simulink model "do_an_tn_ks"  (R2023b)
settings: Solver=VariableStepDiscrete  StartTime=0.0  StopTime=2  MaxStep=1e-7  RelTol=1e-3
values from neighbouring files (symbols this model uses):
  anpha = Vmax^3/(2*Ve*Vmax^2-2*Ve^3)    [daks_delay.m]
  b1 = 2-(wh*Ts1)^2    (= 1.99975325989)    [daks_delay.m]
  b2 = -1    [daks_delay.m]
  b3 = kprv1    [daks_delay.m]
  b4 = kirv1*Ts1+kprv1*((wh*Ts1)^2-2)    [daks_delay.m]
  b5 = kprv1-kirv1*Ts1    [daks_delay.m]
  C = Cmin    [daks_delay.m]
  c1 = 1    [daks_delay.m]
  c2 = kpi+kii*Ts/2    [daks_delay.m]
  c3 = kii*Ts/2-kpi    [daks_delay.m]
  Cf = 20e-6    (= 2e-05)    [daks_delay.m]
  ki1 = Ve/(sqrt(2)*Pe1)    [daks_delay.m]
  ki2 = Ve/(sqrt(2)*Pe2)    [daks_delay.m]
  kv = Vmax/sqrt(2)    [daks_delay.m]
  L = 1.3e-3    (= 0.0013)    [daks_delay.m]
  m4 = (4*m1/Ts^2+2*m2/Ts+m3)/(4*n1/Ts^2+2*n2/Ts+n3)    [daks_delay.m]
  m5 = (-8*m1/Ts^2+2*m3)/(4*n1/Ts^2+2*n2/Ts+n3)    [daks_delay.m]
  m6 = (4*m1/Ts^2-2*m2/Ts+m3)/(4*n1/Ts^2+2*n2/Ts+n3)    [daks_delay.m]
  n5 = -(-8*n1/Ts^2+2*n3)/(4*n1/Ts^2+2*n2/Ts+n3)    [daks_delay.m]
  n6 = -(4*n1/Ts^2-2*n2/Ts+n3)/(4*n1/Ts^2+2*n2/Ts+n3)    [daks_delay.m]
  o = 2*anpha    [daks_delay.m]
  Rf = 0.3    [daks_delay.m]
  sw = 4    [daks_delay.m]
  sw1 = 20    [daks_delay.m]
  Ts = 1/20000    (= 5e-05)    [daks_delay.m]
  Udc = 100    [daks_delay.m]
  wnom = 2*pi*50    (= 314.159265359)    [daks_delay.m]
undefined symbols (not defined in the file or in its folder): den_nz1, den_nz2, DiscIntNeverNeededParam, do_an_tn_ks, Down, i, m, num_nz1, num_nz2, Up
libraries: prociolib x12, peripheralslib x12, spsCurrentMeasurementLib x8, spsIGBTDiodeLib x8, spsSeriesRLCBranchLib x7, simulink x6, spsVoltageMeasurementLib x5, spsBreakerLib x2, simulink_extras x2, spsPowerLib x2, spsDCVoltageSourceLib x2, spsSeriesRLCLoadLib x1
(part 1 of 2)
settings Model: SimulationMode=accelerator  Creator=LEGION  LastModifiedBy=Acer
settings SolverCC: ZeroCrossControl=DisableAll  AlgebraicLoopSolver=TrustRegion
settings DataIOCC: ReturnWorkspaceOutputs=off
settings OptimizationCC: ReuseModelBlockBuffer=off
settings DebuggingCC: UnconnectedInputMsg=warning  UnconnectedOutputMsg=warning  UnconnectedLineMsg=warning
settings ModelReferenceCC: EnableRefExpFcnMdlSchedulingChecks=on
settings SFSimCC: CustomCodeUndefinedFunction=UseInterfaceOnly
settings GRTTargetCC: RTWCAPISignals=on  RTWCAPIParams=on

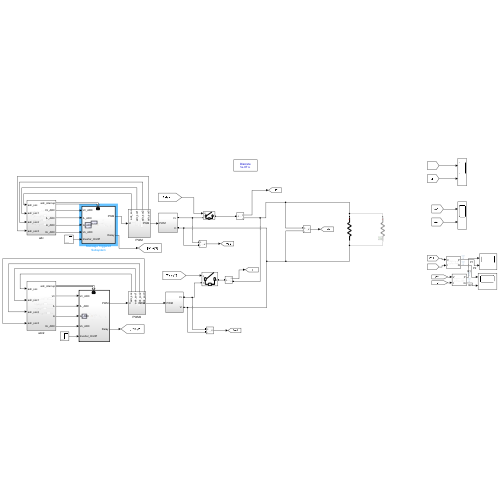
[thumbnail: Simulink's stored preview of the top-level diagram]
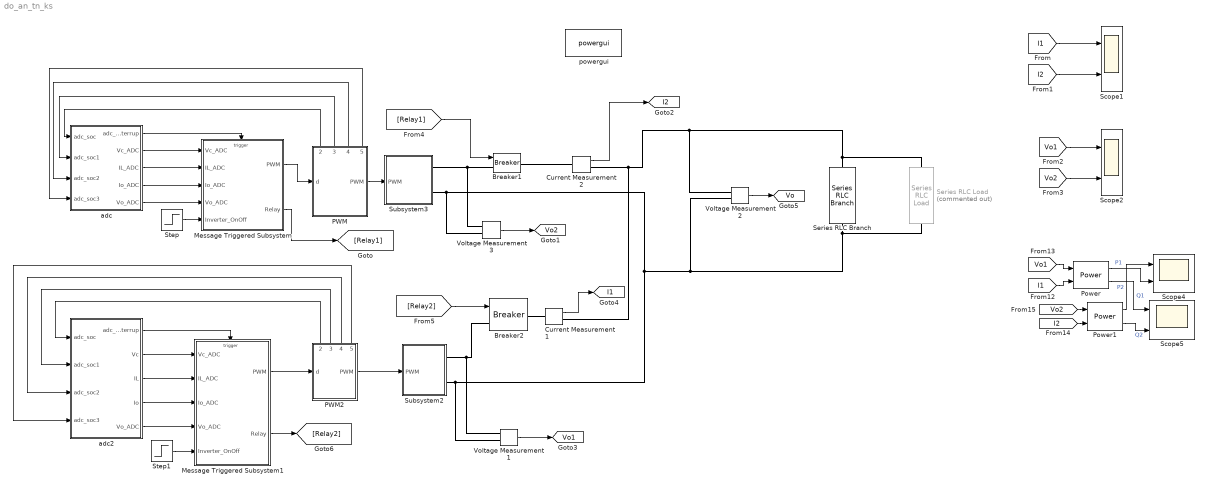
== system do_an_tn_ks ==
  Breaker1 : spsBreakerLib/Breaker  InitialState=0  SwitchingTimes="[1/60  5/60]"  External=on  BreakerResistance=0.01  SnubberResistance=1e6  SnubberCapacitance=inf  Measurements=None  MoreParameters=on  NoBreakLoop=off
  Breaker2 : spsBreakerLib/Breaker  InitialState=0  SwitchingTimes="[1/60  5/60]"  External=on  BreakerResistance=0.01  SnubberResistance=1e6  SnubberCapacitance=inf  Measurements=None  MoreParameters=on  NoBreakLoop=off
  Current Measurement1 : spsCurrentMeasurementLib/Current Measurement  PhasorSimulation=off  OutputType=Complex  PSBequivalent=0
  Current Measurement2 : spsCurrentMeasurementLib/Current Measurement  PhasorSimulation=off  OutputType=Complex  PSBequivalent=0
  Message Triggered Subsystem : Subsystem  InputPortMessageModes=i,i,i,i,i,m  TreatAsAtomicUnit=on
  Message Triggered Subsystem1 : Subsystem  InputPortMessageModes=i,i,i,i,i,m  TreatAsAtomicUnit=on
  PWM : Subsystem
      settings: PortSchema="{\"entries\":[{\"content\":{\"sides\":[{\"content\":{\"connectorIds\":[\"In1\"]},\"type\":\"ConnectorPlacement.EquallySpacedRectSide\",\"uuid\":\"e068b76d-8b58-4347-943a-c1dd0ef851be\"},{\"content\":{\"connectorIds\":[\"Out1\"],\"side\":\"RIGHT\"},\"type\":\"ConnectorPlacement.EquallySpacedRectSide\",\"uuid\":\"70af7750-8974-45f5-ac9e-e83d9d9c07fc\"},{\"content\":{\"connectorIds\":[\"Out2\",\"Out3\",\"Out4\",\"Out5\"],\"side\":\"TOP\"},\"type\":\"ConnectorPlacement.EquallySpacedRectSide\",\"uuid\":\"5d6a6e74-8176-4c49-8c99-236b0d61d046\"}]},\"type\":\"ConnectorPlacement.EquallySpacedConnector\",\"uuid\":\"483dab25-8052-4e69-8bb9-48464924440c\"}],\"packageUris\":[\"http://schema.mathworks.com/mf0/Connector/R2020b\"],\"version\":\"1.0\"}"
  PWM2 : Subsystem
      settings: PortSchema="{\"entries\":[{\"content\":{\"sides\":[{\"content\":{\"connectorIds\":[\"In1\"]},\"type\":\"ConnectorPlacement.EquallySpacedRectSide\",\"uuid\":\"e068b76d-8b58-4347-943a-c1dd0ef851be\"},{\"content\":{\"connectorIds\":[\"Out1\"],\"side\":\"RIGHT\"},\"type\":\"ConnectorPlacement.EquallySpacedRectSide\",\"uuid\":\"70af7750-8974-45f5-ac9e-e83d9d9c07fc\"},{\"content\":{\"connectorIds\":[\"Out2\",\"Out3\",\"Out4\",\"Out5\"],\"side\":\"TOP\"},\"type\":\"ConnectorPlacement.EquallySpacedRectSide\",\"uuid\":\"5d6a6e74-8176-4c49-8c99-236b0d61d046\"}]},\"type\":\"ConnectorPlacement.EquallySpacedConnector\",\"uuid\":\"483dab25-8052-4e69-8bb9-48464924440c\"}],\"packageUris\":[\"http://schema.mathworks.com/mf0/Connector/R2020b\"],\"version\":\"1.0\"}"
  Power : spsPowerLib/Power  Freq=50  Vinit=[1, 0]  Iinit=[1, 0]  Ts=Ts
  Power1 : spsPowerLib/Power  Freq=50  Vinit=[1, 0]  Iinit=[1, 0]  Ts=Ts
  Scope{1..2,4..5} (4 alike) : Scope  NumInputPorts=2
  Series RLC Branch : spsSeriesRLCBranchLib/Series RLC Branch  LConnTagsString=__new0  RConnTagsString=__new0  BranchType=R  Resistance=50  Inductance=1e-3  SetiL0=off  InitialCurrent=0  Capacitance=1e-6  Setx0=off  InitialVoltage=0  Measurements=None
  Series RLC Load : spsSeriesRLCLoadLib/Series RLC Load  Commented=on  LConnTagsString=a  RConnTagsString=__new0  NominalVoltage=220  NominalFrequency=50  ActivePower=3000  InductivePower=0  CapacitivePower=0  Setx0=off  InitialVoltage=0  SetiL0=off  InitialCurrent=0  Measurements=None  LoadType=constant Z
  Step : Step  Time=0.2  SampleTime=0
  Step1 : Step  Time=0.3  SampleTime=0
  Subsystem2 : Subsystem
  Subsystem3 : Subsystem
  Voltage Measurement1 : spsVoltageMeasurementLib/Voltage Measurement  PhasorSimulation=off  OutputType=Complex  PSBequivalent=0
  Voltage Measurement2 : spsVoltageMeasurementLib/Voltage Measurement  PhasorSimulation=off  OutputType=Complex  PSBequivalent=0
  Voltage Measurement3 : spsVoltageMeasurementLib/Voltage Measurement  PhasorSimulation=off  OutputType=Complex  PSBequivalent=0
  adc : Subsystem
  adc2 : Subsystem
  powergui : spspowerguiLib/powergui  Priority=1  SimulationMode=Discrete  SampleTime=1e-7  frequency=60  Iterations=50  frequencyindice=0  Pbase=100e6  ErrMax=1e-4  UnitsV=kV  UnitsW=MW  buscounter=0  FunctionMessages=off  echomessages=off  EnableUseOfTLC=off  CurrentSourceSwitches=off  DisableSnubberDevices=off  DisableRonSwitches=off  DisableVfSwitches=off  DisplayEquations=off  AutomaticDiscreteSolvers=off  SolverType=Tustin/Backward Euler (TBE)  Interpol=off  ExternalGateDelay=off  methode=off  Ts=100  x0status=blocks  SPID=on  SwTol=0  HookPort=off  NonlinearTolerance=1e-4  nMaxIteration=100  ContinueOnMaxIteration=off  RestoreLinks=warning  ResistiveCurrentMeasurement=off  Frange=[0:2:500]  Ylog=off  Xlog=on  ShowGrid=off  save=off  variable=ZData  structure=0  ZoomFFT=off  StartTime=0.0  cycles=1  DisplayStyle=1  fundamental=60  FreqAxis=off  MaxFrequency=1000  frequencyindicesteady=1  RmsSteady=1  display=off
  tag scope: I1=global, I2=global, Vo1=global, Vo2=global, Vo=global
  wires:
  adc/1(adc_interrup) -> Message Triggered Subsystem/Trigger
  PWM/1(PWM) -> Subsystem3/1("PWM ")
  adc/2(Vc_ADC) -> Message Triggered Subsystem/1(Vc_ADC)
  Message Triggered Subsystem/1(PWM) -> PWM/1(d)
  PWM/3(adc_soc1) -> adc/2(adc_soc1)
  PWM/2(adc_soc) -> adc/1(adc_soc)
  Voltage Measurement3/1 -> [Vo2]
  adc/3(IL_ADC) -> Message Triggered Subsystem/2(IL_ADC)
  PWM/4(adc_soc2) -> adc/3(adc_soc2)
  adc/4(Io_ADC) -> Message Triggered Subsystem/3(Io_ADC)
  Voltage Measurement1/1 -> [Vo1]
  PWM2/4(adc_soc2) -> adc2/3(adc_soc2)
  PWM2/2(adc_soc) -> adc2/1(adc_soc)
  PWM2/3(adc_soc1) -> adc2/2(adc_soc1)
  adc2/2(Vc) -> Message Triggered Subsystem1/1(Vc_ADC)
  PWM2/1(PWM) -> Subsystem2/1("PWM ")
  adc2/1(adc_interrup) -> Message Triggered Subsystem1/Trigger
  Current Measurement2/1 -> [I2]
  Current Measurement1/1 -> [I1]
  [I1] -> Scope1/1
  [I2] -> Scope1/2
  Step/1 -> Message Triggered Subsystem/5(Inverter_OnOff)
  [Vo1] -> Scope2/1
  [Vo2] -> Scope2/2
  Voltage Measurement2/1 -> [Vo]
  PWM/5(adc_soc3) -> adc/4(adc_soc3)
  adc/5(Vo_ADC) -> Message Triggered Subsystem/4(Vo_ADC)
  Power/1 -> Scope4/2  "P1"
  [Vo1] -> Power/1
  Power/2 -> Scope5/1  "Q1"
  Power1/2 -> Scope5/2  "Q2"
  [I2] -> Power1/2
  [I1] -> Power/2
  Power1/1 -> Scope4/1  "P2"
  [Vo2] -> Power1/1
  Message Triggered Subsystem1/1(PWM) -> PWM2/1(d)
  adc2/3(IL) -> Message Triggered Subsystem1/2(IL_ADC)
  adc2/4(Io) -> Message Triggered Subsystem1/3(Io_ADC)
  PWM2/5(adc_soc3) -> adc2/4(adc_soc3)
  adc2/5(Vo_ADC) -> Message Triggered Subsystem1/4(Vo_ADC)
  Step1/1 -> Message Triggered Subsystem1/5(Inverter_OnOff)
  Message Triggered Subsystem/2(Relay) -> [Relay1]
  [Relay1] -> Breaker1/1
  Message Triggered Subsystem1/2(Relay) -> [Relay2]
  [Relay2] -> Breaker2/1
  connections:
  Voltage Measurement3/LConn2 -- Subsystem3/RConn2 -- Series RLC Load/RConn1 -- Series RLC Branch/RConn1 -- Voltage Measurement2/LConn2 -- Voltage Measurement1/LConn2 -- Subsystem2/RConn2
  Breaker1/LConn1 -- Voltage Measurement3/LConn1 -- Subsystem3/RConn1
  Breaker1/RConn1 -- Current Measurement2/LConn1
  Current Measurement1/RConn1 -- Series RLC Branch/LConn1 -- Series RLC Load/LConn1 -- Voltage Measurement2/LConn1 -- Current Measurement2/RConn1
  Breaker2/RConn1 -- Current Measurement1/LConn1
  Breaker2/LConn1 -- Voltage Measurement1/LConn1 -- Subsystem2/RConn1

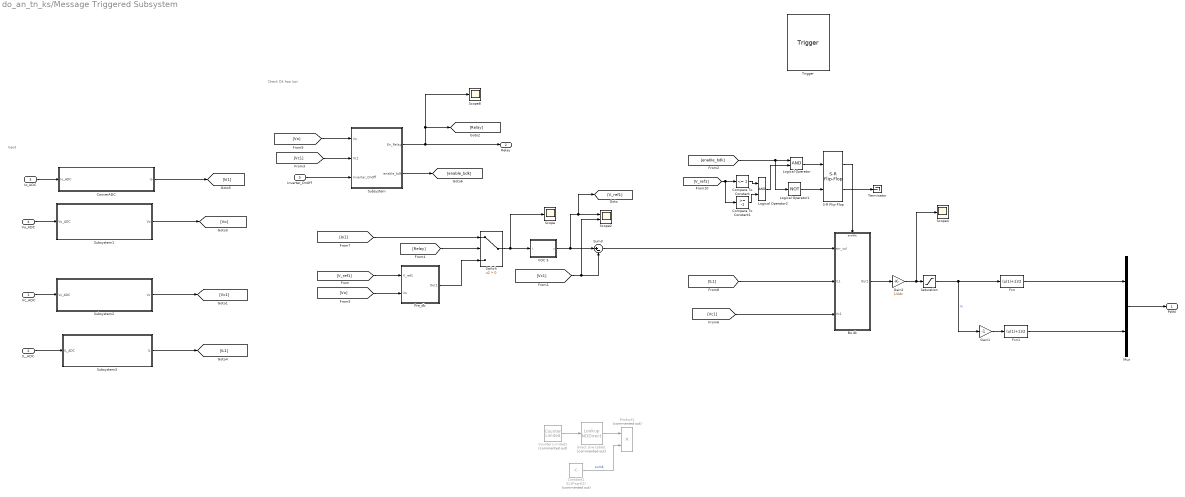
== system do_an_tn_ks/Message Triggered Subsystem ==
  note: Check Dk hoa luoi
  note: Input
  Vc_ADC : Inport
  IL_ADC : Inport  Port=2
  Io_ADC : Inport  Port=3
  Vo_ADC : Inport  Port=4
  Inverter_OnOff : Inport  Port=5
  Trigger : TriggerPort  TriggerType=message  ScheduleAsAperiodic=off  FunctionName=MessageTriggeredSubsystem  FunctionVisibility=scoped  VariantControl=(inherit)  PortDimensions=1
  Bo dk : Subsystem
  Compare To Constant : simulink/Logic and Bit Operations/Compare To Constant  relop=<=  const=1  OutDataTypeStr=boolean
  Compare To Constant1 : simulink/Logic and Bit Operations/Compare To Constant  relop=>=  const=-1  OutDataTypeStr=boolean
  Constant1 : Constant  Commented=on  Value=51.8*sqrt(2)  OutDataTypeStr=single  SampleTime=-1
  ConverADC : Subsystem
  Counter Limited1 : simulink/Sources/Counter Limited  Commented=on  uplimit=399  tsamp=-1
  Fcn : Fcn  Expr=(u(1)+1)/2
  Fcn1 : Fcn  Expr=(u(1)+1)/2
  Gain1 : Gain  Gain=-1
  Gain2 : Gain  Gain=1/Udc
  Logical Operator : Logic  AllPortsSameDT=off  OutDataTypeStr=boolean
  Logical Operator1 : Logic  Operator=NOT  AllPortsSameDT=off  OutDataTypeStr=boolean
  Logical Operator2 : Logic  AllPortsSameDT=off  OutDataTypeStr=boolean
  Mux : Mux  Inputs=2
  Pre_db : Subsystem
  Product1 : Product  Commented=on
  S-R Flip-Flop : simulink_extras/Flip Flops/S-R Flip-Flop  initial_condition=0
  Saturation : Saturate  UpperLimit=1  LowerLimit=-1
  Scope : Scope
  Scope2 : Scope  NumInputPorts=2
  Scope4 : Scope
  Scope8 : Scope
  Subsystem : Subsystem
  Subsystem1 : Subsystem
  Subsystem2 : Subsystem
  Subsystem3 : Subsystem
  Sum3 : Sum  Inputs=|+-
  Switch : Switch  Criteria=u2 > Threshold  SaturateOnIntegerOverflow=off  InputSameDT=off
  Terminator : Terminator
  VOC 3 : Subsystem
  direct sine table1 : LookupNDDirect  Commented=on  NumberOfTableDimensions=1  Table=sin( 2*pi *50* (0:399)/20000)'  TableDataTypeStr=single
  PWM : Outport
  Relay : Outport  Port=2
  wires:
  Constant1/1 -> Product1/2  "sum6"
  direct sine table1/1 -> Product1/1
  Sum3/1 -> Bo dk/1(err_vol)
  Saturation/1 -> Fcn/1, Gain1/1  "m"
  Gain1/1 -> Fcn1/1
  Gain2/1 -> Scope4/1, Saturation/1
  Counter Limited1/1 -> direct sine table1/1
  Mux/1 -> PWM/1
  Fcn/1 -> Mux/1
  Fcn1/1 -> Mux/2
  VOC 3/1(v) -> [V_ref1], Scope2/1, Sum3/1
  Switch/1 -> Scope/1, VOC 3/1(i)
  [Relay] -> Switch/2
  [Vc1] -> Scope2/2, Sum3/2
  [Vo] -> Subsystem/1(Vo)
  [Vc1] -> Subsystem/2(Vc1)
  Inverter_OnOff/1 -> Subsystem/3(Inverter_OnOff)
  Subsystem/1(En_Relay) -> Scope8/1, [Relay], Relay/1
  Io_ADC/1 -> ConverADC/1(Io_ADC)
  Subsystem1/1(Vo) -> [Vo]
  Vo_ADC/1 -> Subsystem1/1(Vo_ADC)
  Vc_ADC/1 -> Subsystem2/1(Vc_ADC)
  Subsystem2/1(Vc) -> [Vc1]
  IL_ADC/1 -> Subsystem3/1(IL_ADC)
  Subsystem3/1(IL) -> [IL1]
  [V_ref1] -> Pre_db/1(V_ref1)
  [Vo] -> Pre_db/2(Vo)
  Pre_db/1(Out1) -> Switch/3
  ConverADC/1(Io) -> [Io1]
  [Io1] -> Switch/1
  [IL1] -> Bo dk/2(IL1)
  [Vc1] -> Bo dk/3(Vc1)
  Bo dk/1(Out1) -> Gain2/1
  Subsystem/2(enable_bdk) -> [enable_bdk]
  Logical Operator1/1 -> S-R Flip-Flop/2
  S-R Flip-Flop/2 -> Terminator/1
  S-R Flip-Flop/1 -> Bo dk/Enable
  Logical Operator/1 -> S-R Flip-Flop/1
  [enable_bdk] -> Logical Operator1/1, Logical Operator/1
  [V_ref1] -> Compare To Constant1/1, Compare To Constant/1
  Compare To Constant/1 -> Logical Operator2/1
  Compare To Constant1/1 -> Logical Operator2/2
  Logical Operator2/1 -> Logical Operator/2

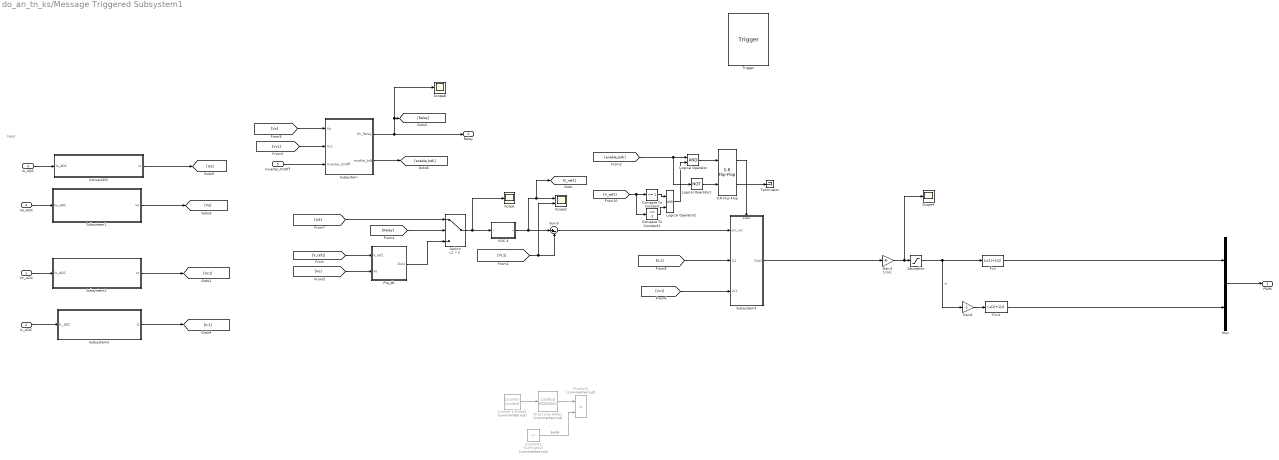
== system do_an_tn_ks/Message Triggered Subsystem1 ==
  note: Input
  Vc_ADC : Inport
  IL_ADC : Inport  Port=2
  Io_ADC : Inport  Port=3
  Vo_ADC : Inport  Port=4
  Inverter_OnOff : Inport  Port=5
  Trigger : TriggerPort  TriggerType=message  ScheduleAsAperiodic=off  FunctionName=MessageTriggeredSubsystem1  FunctionVisibility=scoped  VariantControl=(inherit)  PortDimensions=1
  Compare To Constant : simulink/Logic and Bit Operations/Compare To Constant  relop=<=  const=1  OutDataTypeStr=boolean
  Compare To Constant1 : simulink/Logic and Bit Operations/Compare To Constant  relop=>=  const=-1  OutDataTypeStr=boolean
  Constant1 : Constant  Commented=on  Value=51.8*sqrt(2)  OutDataTypeStr=single  SampleTime=-1
  ConverADC : Subsystem
  Counter Limited1 : simulink/Sources/Counter Limited  Commented=on  uplimit=399  tsamp=-1
  Fcn : Fcn  Expr=(u(1)+1)/2
  Fcn1 : Fcn  Expr=(u(1)+1)/2
  Gain1 : Gain  Gain=-1
  Gain2 : Gain  Gain=1/Udc
  Logical Operator : Logic  AllPortsSameDT=off  OutDataTypeStr=boolean
  Logical Operator1 : Logic  Operator=NOT  AllPortsSameDT=off  OutDataTypeStr=boolean
  Logical Operator2 : Logic  AllPortsSameDT=off  OutDataTypeStr=boolean
  Mux : Mux  Inputs=2
  Pre_db : Subsystem
  Product1 : Product  Commented=on
  S-R Flip-Flop : simulink_extras/Flip Flops/S-R Flip-Flop  initial_condition=0
  Saturation : Saturate  UpperLimit=1  LowerLimit=-1
  Scope : Scope
  Scope2 : Scope  NumInputPorts=2
  Scope4 : Scope
  Scope8 : Scope
  Subsystem : Subsystem
  Subsystem1 : Subsystem
  Subsystem2 : Subsystem
  Subsystem3 : Subsystem
  Subsystem4 : Subsystem
  Sum3 : Sum  Inputs=|+-
  Switch : Switch  Criteria=u2 > Threshold  SaturateOnIntegerOverflow=off  InputSameDT=off
  Terminator : Terminator
  VOC 3 : Subsystem
  direct sine table1 : LookupNDDirect  Commented=on  NumberOfTableDimensions=1  Table=sin( 2*pi *50* (0:399)/20000)'  TableDataTypeStr=single
  PWM : Outport
  Relay : Outport  Port=2
  wires:
  Subsystem/2(enable_bdk) -> [enable_bdk]
  Subsystem4/1(Out1) -> Gain2/1
  [Vc1] -> Subsystem4/3(Vc1)
  [IL1] -> Subsystem4/2(IL1)
  [Io1] -> Switch/1
  ConverADC/1(Io) -> [Io1]
  Pre_db/1(Out1) -> Switch/3
  [Vo] -> Pre_db/2(Vo)
  [V_ref1] -> Pre_db/1(V_ref1)
  Subsystem3/1(IL) -> [IL1]
  IL_ADC/1 -> Subsystem3/1(IL_ADC)
  Subsystem2/1(Vc) -> [Vc1]
  Vc_ADC/1 -> Subsystem2/1(Vc_ADC)
  Vo_ADC/1 -> Subsystem1/1(Vo_ADC)
  Subsystem1/1(Vo) -> [Vo]
  Io_ADC/1 -> ConverADC/1(Io_ADC)
  Subsystem/1(En_Relay) -> Relay/1, [Relay], Scope8/1
  Inverter_OnOff/1 -> Subsystem/3(Inverter_OnOff)
  [Vc1] -> Subsystem/2(Vc1)
  [Vo] -> Subsystem/1(Vo)
  [Vc1] -> Sum3/2, Scope2/2
  [Relay] -> Switch/2
  Switch/1 -> VOC 3/1(i), Scope/1
  VOC 3/1(v) -> Sum3/1, Scope2/1, [V_ref1]
  Fcn1/1 -> Mux/2
  Fcn/1 -> Mux/1
  Mux/1 -> PWM/1
  Counter Limited1/1 -> direct sine table1/1
  Gain2/1 -> Saturation/1, Scope4/1
  Gain1/1 -> Fcn1/1
  Saturation/1 -> Gain1/1, Fcn/1  "m"
  Sum3/1 -> Subsystem4/1(err_vol)
  direct sine table1/1 -> Product1/1
  Constant1/1 -> Product1/2  "sum6"
  [enable_bdk] -> Logical Operator1/1, Logical Operator/1
  Logical Operator2/1 -> Logical Operator/2
  Logical Operator/1 -> S-R Flip-Flop/1
  S-R Flip-Flop/1 -> Subsystem4/Enable
  Logical Operator1/1 -> S-R Flip-Flop/2
  S-R Flip-Flop/2 -> Terminator/1
  Compare To Constant1/1 -> Logical Operator2/2
  Compare To Constant/1 -> Logical Operator2/1
  [V_ref1] -> Compare To Constant1/1, Compare To Constant/1

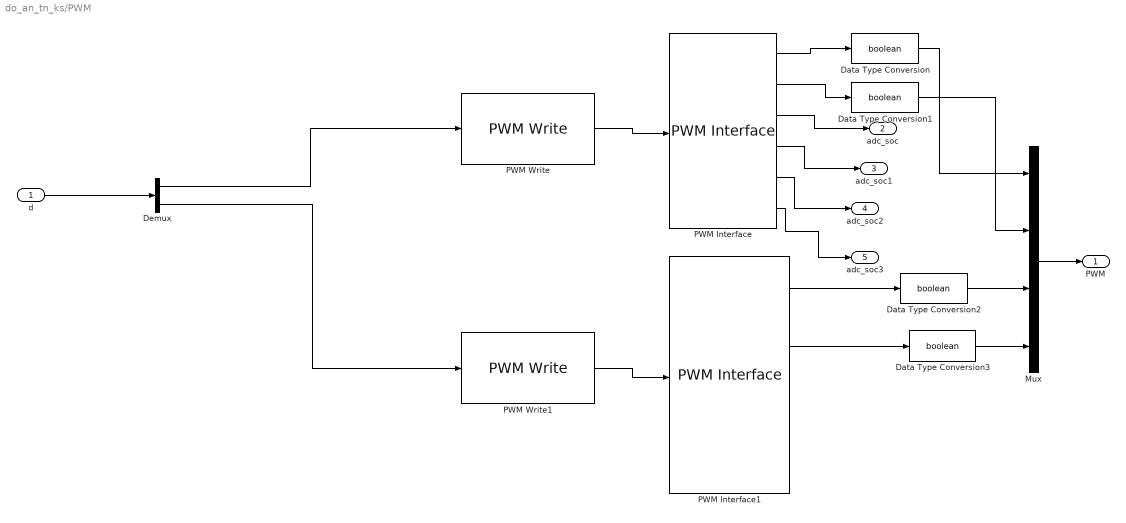
== system do_an_tn_ks/PWM ==
  d : Inport
  Data Type Conversion{,1..3} (4 alike) : DataTypeConversion  OutDataTypeStr=boolean  SaturateOnIntegerOverflow=off  RndMeth=Floor
  Demux : Demux  Outputs=2
  Mux : Mux
  PWM Interface : peripheralslib/PWM Interface  Period=1/10e3  OutSigMode=Switching  CounterMode=Up-Down  GenCompPWM=on  DeadTimeTopPWM=2e-6  DeadTimeBottomPWM=2e-6  EventCondition2=End of PWM period  DataType=single  PWMAtStartPeriod=High  PWMAtMidPeriod=NoChange  PWMAtCMP1=Low  PWMAtCMP1UpCnt=Low  PWMAtCMP1DwnCnt=High  PWMAtCMP2=NoChange  PWMAtCMP2UpCnt=NoChange  PWMAtCMP2DwnCnt=NoChange  OutCountDir=off  PhaseOffset=0  EventType=ADC start  EventCondition1=Mid or End of PWM period  NumADCSOCToWait=1st event  NumADCSOCReplica=4  InterruptCond=End of PWM period  IntLatency=0  NumInterruptToWait=1st event
      settings: SamplingMode=Mid or End of PWM period
  PWM Interface1 : peripheralslib/PWM Interface  Period=1/10e3  OutSigMode=Switching  CounterMode=Up-Down  GenCompPWM=on  DeadTimeTopPWM=2e-6  DeadTimeBottomPWM=2e-6  EventCondition2=End of PWM period  DataType=single  PWMAtStartPeriod=High  PWMAtMidPeriod=NoChange  PWMAtCMP1=Low  PWMAtCMP1UpCnt=Low  PWMAtCMP1DwnCnt=High  PWMAtCMP2=NoChange  PWMAtCMP2UpCnt=NoChange  PWMAtCMP2DwnCnt=NoChange  OutCountDir=off  PhaseOffset=0  EventType=ADC start  EventCondition1=Mid of PWM period  NumADCSOCToWait=1st event  NumADCSOCReplica=2  InterruptCond=End of PWM period  IntLatency=0  NumInterruptToWait=1st event
      settings: SamplingMode=Mid or End of PWM period
  PWM Write : prociolib/PWM Write  ShowPeriodInp=off  ShowPhaseInp=off  PeripheralConfigBtnCtrl=0  BlockSID=do_an_tn_ks:3474
  PWM Write1 : prociolib/PWM Write  ShowPeriodInp=off  ShowPhaseInp=off  PeripheralConfigBtnCtrl=0  BlockSID=do_an_tn_ks:3475
  PWM : Outport
  adc_soc : Outport  Port=2
  adc_soc1 : Outport  Port=3
  adc_soc2 : Outport  Port=4
  adc_soc3 : Outport  Port=5
  wires:
  PWM Write1/1 -> PWM Interface1/1
  Data Type Conversion1/1 -> Mux/2
  PWM Write/1 -> PWM Interface/1
  PWM Interface/2 -> Data Type Conversion1/1
  Mux/1 -> PWM/1
  Demux/2 -> PWM Write1/1
  PWM Interface/1 -> Data Type Conversion/1
  Data Type Conversion2/1 -> Mux/3
  Data Type Conversion3/1 -> Mux/4
  PWM Interface1/2 -> Data Type Conversion3/1
  Data Type Conversion/1 -> Mux/1
  PWM Interface1/1 -> Data Type Conversion2/1
  Demux/1 -> PWM Write/1
  d/1 -> Demux/1
  PWM Interface/3 -> adc_soc/1
  PWM Interface/4 -> adc_soc1/1
  PWM Interface/5 -> adc_soc2/1
  PWM Interface/6 -> adc_soc3/1

== system do_an_tn_ks/PWM2 ==
  d : Inport
  Data Type Conversion{,1..3} (4 alike) : DataTypeConversion  OutDataTypeStr=boolean  SaturateOnIntegerOverflow=off  RndMeth=Floor
  Demux : Demux  Outputs=2
  Mux : Mux
  PWM Interface : peripheralslib/PWM Interface  Period=1/10e3  OutSigMode=Switching  CounterMode=Up-Down  GenCompPWM=on  DeadTimeTopPWM=2e-6  DeadTimeBottomPWM=2e-6  EventCondition2=End of PWM period  DataType=single  PWMAtStartPeriod=High  PWMAtMidPeriod=NoChange  PWMAtCMP1=Low  PWMAtCMP1UpCnt=Low  PWMAtCMP1DwnCnt=High  PWMAtCMP2=NoChange  PWMAtCMP2UpCnt=NoChange  PWMAtCMP2DwnCnt=NoChange  OutCountDir=off  PhaseOffset=0  EventType=ADC start  EventCondition1=Mid or End of PWM period  NumADCSOCToWait=1st event  NumADCSOCReplica=4  InterruptCond=End of PWM period  IntLatency=0  NumInterruptToWait=1st event
      settings: SamplingMode=Mid or End of PWM period
  PWM Interface1 : peripheralslib/PWM Interface  Period=1/10e3  OutSigMode=Switching  CounterMode=Up-Down  GenCompPWM=on  DeadTimeTopPWM=2e-6  DeadTimeBottomPWM=2e-6  EventCondition2=End of PWM period  DataType=single  PWMAtStartPeriod=High  PWMAtMidPeriod=NoChange  PWMAtCMP1=Low  PWMAtCMP1UpCnt=Low  PWMAtCMP1DwnCnt=High  PWMAtCMP2=NoChange  PWMAtCMP2UpCnt=NoChange  PWMAtCMP2DwnCnt=NoChange  OutCountDir=off  PhaseOffset=0  EventType=ADC start  EventCondition1=Mid of PWM period  NumADCSOCToWait=1st event  NumADCSOCReplica=2  InterruptCond=End of PWM period  IntLatency=0  NumInterruptToWait=1st event
      settings: SamplingMode=Mid or End of PWM period
  PWM Write : prociolib/PWM Write  ShowPeriodInp=off  ShowPhaseInp=off  PeripheralConfigBtnCtrl=0  BlockSID=do_an_tn_ks:3847
  PWM Write1 : prociolib/PWM Write  ShowPeriodInp=off  ShowPhaseInp=off  PeripheralConfigBtnCtrl=0  BlockSID=do_an_tn_ks:3848
  PWM : Outport
  adc_soc : Outport  Port=2
  adc_soc1 : Outport  Port=3
  adc_soc2 : Outport  Port=4
  adc_soc3 : Outport  Port=5
  wires:
  PWM Interface/5 -> adc_soc2/1
  PWM Interface/4 -> adc_soc1/1
  PWM Interface/3 -> adc_soc/1
  d/1 -> Demux/1
  Demux/1 -> PWM Write/1
  PWM Interface1/1 -> Data Type Conversion2/1
  Data Type Conversion/1 -> Mux/1
  PWM Interface1/2 -> Data Type Conversion3/1
  Data Type Conversion3/1 -> Mux/4
  Data Type Conversion2/1 -> Mux/3
  PWM Interface/1 -> Data Type Conversion/1
  Demux/2 -> PWM Write1/1
  Mux/1 -> PWM/1
  PWM Interface/2 -> Data Type Conversion1/1
  PWM Write/1 -> PWM Interface/1
  Data Type Conversion1/1 -> Mux/2
  PWM Write1/1 -> PWM Interface1/1
  PWM Interface/6 -> adc_soc3/1

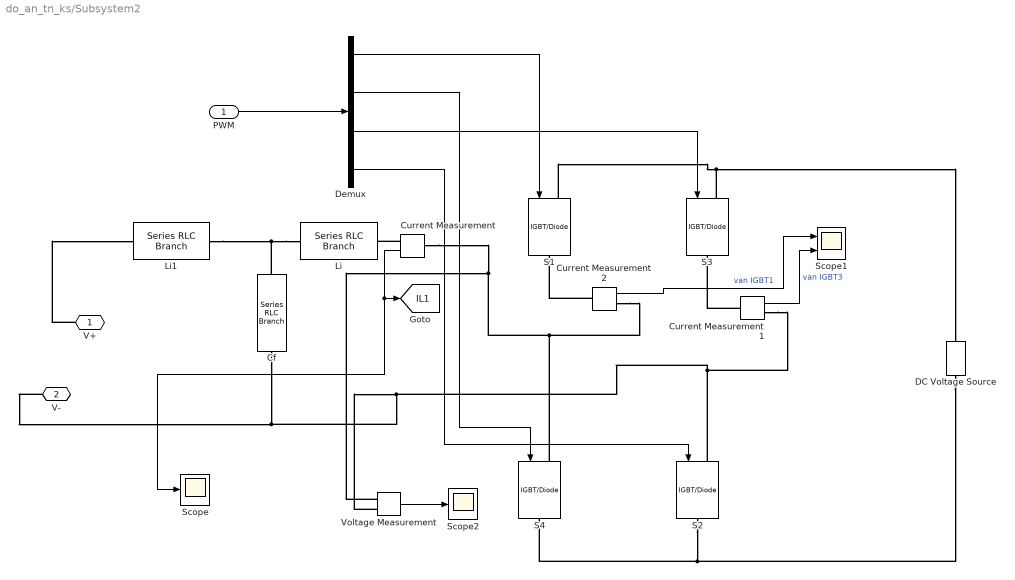
== system do_an_tn_ks/Subsystem2 ==
  "PWM " : Inport
  "   Cf" : spsSeriesRLCBranchLib/Series RLC Branch  LConnTagsString=__new0  RConnTagsString=__new0  BranchType=C  Resistance=0.1  Inductance=1e-3  SetiL0=off  InitialCurrent=0  Capacitance=Cf  Setx0=off  InitialVoltage=0  Measurements=None
  Current Measurement : spsCurrentMeasurementLib/Current Measurement  PhasorSimulation=off  OutputType=Complex  PSBequivalent=0
  Current Measurement1 : spsCurrentMeasurementLib/Current Measurement  PhasorSimulation=off  OutputType=Complex  PSBequivalent=0
  Current Measurement2 : spsCurrentMeasurementLib/Current Measurement  PhasorSimulation=off  OutputType=Complex  PSBequivalent=0
  DC Voltage Source : spsDCVoltageSourceLib/DC Voltage Source  Amplitude=Udc  Measurements=None
  Demux : Demux
  Li : spsSeriesRLCBranchLib/Series RLC Branch  LConnTagsString=__new0  RConnTagsString=__new0  BranchType=RL  Resistance=Rf  Inductance=L  SetiL0=off  InitialCurrent=0  Capacitance=1e-6  Setx0=off  InitialVoltage=0  Measurements=None
  Li1 : spsSeriesRLCBranchLib/Series RLC Branch  LConnTagsString=__new0  RConnTagsString=__new0  BranchType=L  Resistance=Rf  Inductance=470e-6  SetiL0=off  InitialCurrent=0  Capacitance=1e-6  Setx0=off  InitialVoltage=0  Measurements=None
  S{1..4} (4 alike) : spsIGBTDiodeLib/IGBT//Diode  Ron=0.001  Rs=1e5  Cs=inf  Measurements=off
  Scope : Scope
  Scope1 : Scope  NumInputPorts=2
  Scope2 : Scope
  Voltage Measurement : spsVoltageMeasurementLib/Voltage Measurement  PhasorSimulation=off  OutputType=Complex  PSBequivalent=0
  V+ : PMIOPort  Side=Right
  V- : PMIOPort  Port=2  Side=Right
  tag scope: IL1=global
  wires:
  Demux/4 -> S2/1
  Demux/3 -> S3/1
  Demux/2 -> S4/1
  Current Measurement2/1 -> Scope1/1  "van IGBT1"
  Voltage Measurement/1 -> Scope2/1
  Current Measurement1/1 -> Scope1/2  "van IGBT3"
  Current Measurement/1 -> [IL1], Scope/1
  Demux/1 -> S1/1
  "PWM "/1 -> Demux/1
  connections:
  Current Measurement2/LConn1 -- S1/RConn1
  Current Measurement1/LConn1 -- S3/RConn1
  Current Measurement/RConn1 -- Li/RConn1
  S4/RConn1 -- DC Voltage Source/LConn1 -- S2/RConn1
  "   Cf"/RConn1 -- V-/RConn1 -- Voltage Measurement/LConn2 -- Current Measurement1/RConn1 -- S2/LConn1
  S3/LConn1 -- S1/LConn1 -- DC Voltage Source/RConn1
  Current Measurement/LConn1 -- Voltage Measurement/LConn1 -- Current Measurement2/RConn1 -- S4/LConn1
  Li/LConn1 -- Li1/RConn1 -- "   Cf"/LConn1
  V+/RConn1 -- Li1/LConn1

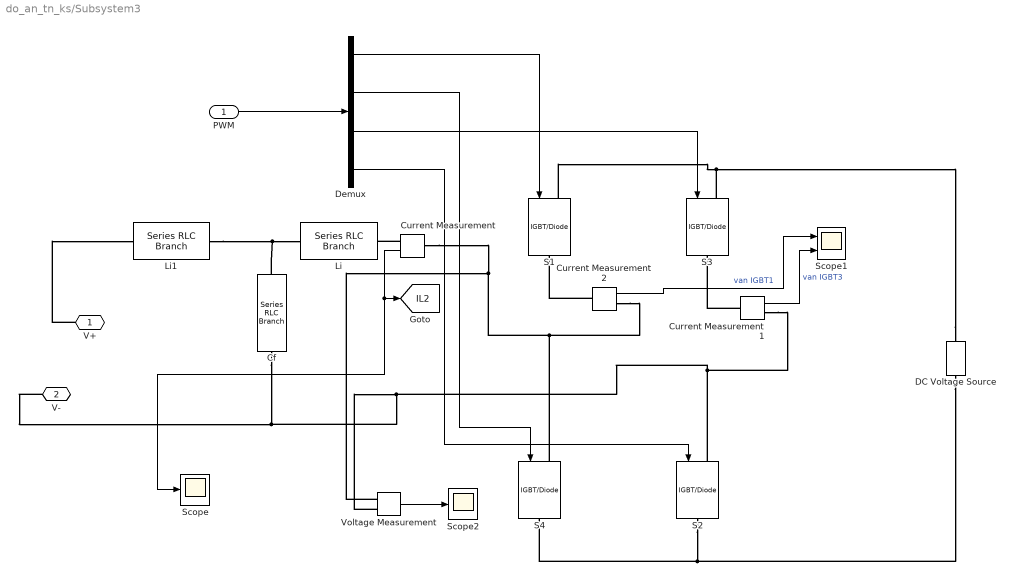
== system do_an_tn_ks/Subsystem3 ==
  "PWM " : Inport
  "   Cf" : spsSeriesRLCBranchLib/Series RLC Branch  LConnTagsString=__new0  RConnTagsString=__new0  BranchType=C  Resistance=0.1  Inductance=1e-3  SetiL0=off  InitialCurrent=0  Capacitance=Cf  Setx0=off  InitialVoltage=0  Measurements=None
  Current Measurement : spsCurrentMeasurementLib/Current Measurement  PhasorSimulation=off  OutputType=Complex  PSBequivalent=0
  Current Measurement1 : spsCurrentMeasurementLib/Current Measurement  PhasorSimulation=off  OutputType=Complex  PSBequivalent=0
  Current Measurement2 : spsCurrentMeasurementLib/Current Measurement  PhasorSimulation=off  OutputType=Complex  PSBequivalent=0
  DC Voltage Source : spsDCVoltageSourceLib/DC Voltage Source  Amplitude=Udc  Measurements=None
  Demux : Demux
  Li : spsSeriesRLCBranchLib/Series RLC Branch  LConnTagsString=__new0  RConnTagsString=__new0  BranchType=RL  Resistance=Rf  Inductance=L  SetiL0=off  InitialCurrent=0  Capacitance=1e-6  Setx0=off  InitialVoltage=0  Measurements=None
  Li1 : spsSeriesRLCBranchLib/Series RLC Branch  LConnTagsString=__new0  RConnTagsString=__new0  BranchType=L  Resistance=Rf  Inductance=470e-6  SetiL0=off  InitialCurrent=0  Capacitance=1e-6  Setx0=off  InitialVoltage=0  Measurements=None
  S{1..4} (4 alike) : spsIGBTDiodeLib/IGBT//Diode  Ron=0.001  Rs=1e5  Cs=inf  Measurements=off
  Scope : Scope
  Scope1 : Scope  NumInputPorts=2
  Scope2 : Scope
  Voltage Measurement : spsVoltageMeasurementLib/Voltage Measurement  PhasorSimulation=off  OutputType=Complex  PSBequivalent=0
  V+ : PMIOPort  Side=Right
  V- : PMIOPort  Port=2  Side=Right
  tag scope: IL2=global
  wires:
  "PWM "/1 -> Demux/1
  Demux/1 -> S1/1
  Current Measurement/1 -> Scope/1, [IL2]
  Current Measurement1/1 -> Scope1/2  "van IGBT3"
  Voltage Measurement/1 -> Scope2/1
  Current Measurement2/1 -> Scope1/1  "van IGBT1"
  Demux/2 -> S4/1
  Demux/3 -> S3/1
  Demux/4 -> S2/1
  connections:
  V+/RConn1 -- Li1/LConn1
  S4/LConn1 -- Current Measurement2/RConn1 -- Voltage Measurement/LConn1 -- Current Measurement/LConn1
  DC Voltage Source/RConn1 -- S1/LConn1 -- S3/LConn1
  S2/LConn1 -- Current Measurement1/RConn1 -- Voltage Measurement/LConn2 -- V-/RConn1 -- "   Cf"/RConn1
  S2/RConn1 -- DC Voltage Source/LConn1 -- S4/RConn1
  Current Measurement/RConn1 -- Li/RConn1
  Current Measurement1/LConn1 -- S3/RConn1
  Current Measurement2/LConn1 -- S1/RConn1
  Li1/RConn1 -- "   Cf"/LConn1 -- Li/LConn1

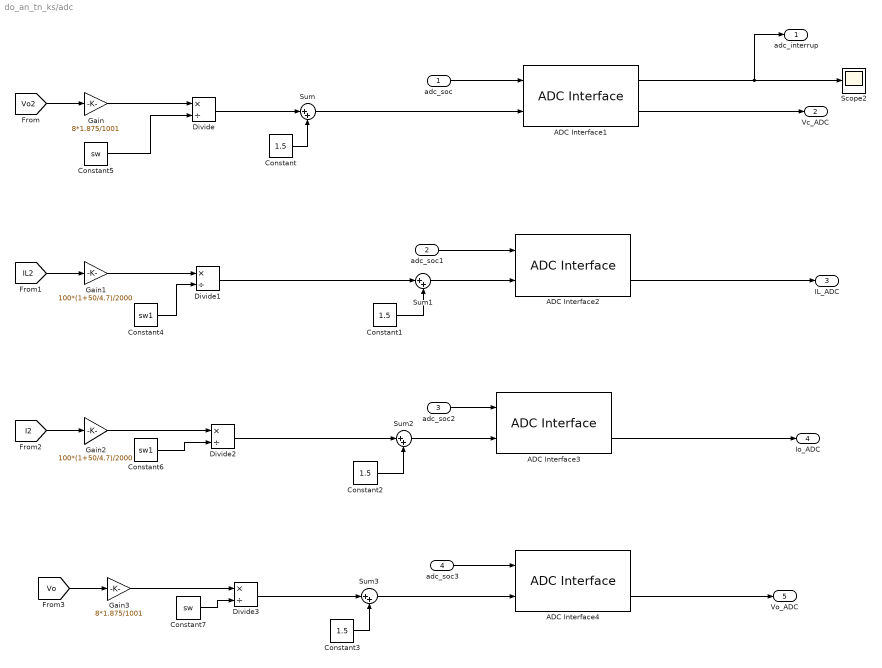
== system do_an_tn_ks/adc ==
  adc_soc : Inport
  adc_soc1 : Inport  Port=2
  adc_soc2 : Inport  Port=3
  adc_soc3 : Inport  Port=4
  ADC Interface{1..4} (4 alike) : peripheralslib/ADC Interface  ADCResolution=12  HighVref=3.3  AcqTime=15*1/(40e6)  ConvTime=12*1/(40e6)  TimeConstant=0  SoftTrig=off  SampleTime=1e-3  NumCh=1  ConvType=Sequential  EnInterrupt=on  IntCondition=Acquisition + Conversion time  EnWatchdog=off  LowThreshold=.1  HighThreshold=2.9  IntLatency=0
  Constant{,1..3} (4 alike) : Constant  Value=1.5
  Constant4 : Constant  Value=sw1
  Constant5 : Constant  Value=sw
  Constant6 : Constant  Value=sw1
  Constant7 : Constant  Value=sw
  Divide{,1..3} (4 alike) : Product  Inputs=*/
  Gain : Gain  Gain=8*1.875/1001
  Gain1 : Gain  Gain=100*(1+50/4.7)/2000
  Gain2 : Gain  Gain=100*(1+50/4.7)/2000
  Gain3 : Gain  Gain=8*1.875/1001
  Scope2 : Scope
  Sum{,1..3} (4 alike) : Sum  Inputs=|++
  adc_interrup : Outport
  Vc_ADC : Outport  Port=2
  IL_ADC : Outport  Port=3
  Io_ADC : Outport  Port=4
  Vo_ADC : Outport  Port=5
  wires:
  adc_soc/1 -> ADC Interface1/1
  [Vo2] -> Gain/1
  Constant/1 -> Sum/2
  Sum/1 -> ADC Interface1/2
  ADC Interface1/2 -> Vc_ADC/1
  adc_soc1/1 -> ADC Interface2/1
  [IL2] -> Gain1/1
  Sum1/1 -> ADC Interface2/2
  Constant1/1 -> Sum1/2
  ADC Interface1/1 -> adc_interrup/1, Scope2/1
  ADC Interface2/2 -> IL_ADC/1
  [I2] -> Gain2/1
  Constant2/1 -> Sum2/2
  ADC Interface3/2 -> Io_ADC/1
  adc_soc2/1 -> ADC Interface3/1
  Sum2/1 -> ADC Interface3/2
  Constant3/1 -> Sum3/2
  [Vo] -> Gain3/1
  adc_soc3/1 -> ADC Interface4/1
  Sum3/1 -> ADC Interface4/2
  ADC Interface4/2 -> Vo_ADC/1
  Gain/1 -> Divide/1
  Divide/1 -> Sum/1
  Gain1/1 -> Divide1/1
  Divide1/1 -> Sum1/1
  Divide2/1 -> Sum2/1
  Gain2/1 -> Divide2/1
  Gain3/1 -> Divide3/1
  Divide3/1 -> Sum3/1
  Constant5/1 -> Divide/2
  Constant4/1 -> Divide1/2
  Constant6/1 -> Divide2/2
  Constant7/1 -> Divide3/2

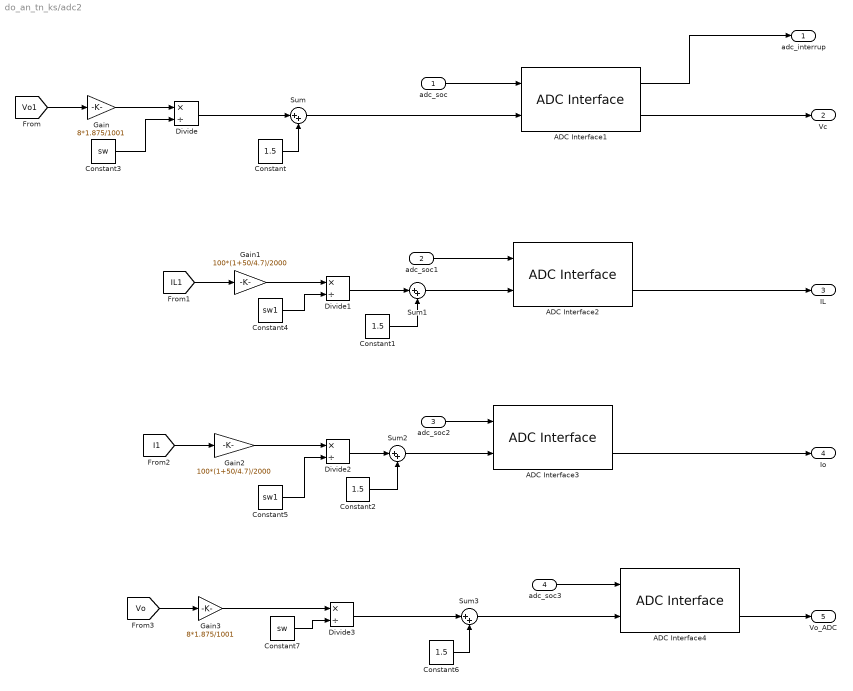
== system do_an_tn_ks/adc2 ==
  adc_soc : Inport
  adc_soc1 : Inport  Port=2
  adc_soc2 : Inport  Port=3
  adc_soc3 : Inport  Port=4
  ADC Interface{1..4} (4 alike) : peripheralslib/ADC Interface  ADCResolution=12  HighVref=3.3  AcqTime=15*1/(40e6)  ConvTime=12*1/(40e6)  TimeConstant=0  SoftTrig=off  SampleTime=1e-3  NumCh=1  ConvType=Sequential  EnInterrupt=on  IntCondition=Acquisition + Conversion time  EnWatchdog=off  LowThreshold=.1  HighThreshold=2.9  IntLatency=0
  Constant{,1..2,6} (4 alike) : Constant  Value=1.5
  Constant3 : Constant  Value=sw
  Constant4 : Constant  Value=sw1
  Constant5 : Constant  Value=sw1
  Constant7 : Constant  Value=sw
  Divide{,1..3} (4 alike) : Product  Inputs=*/
  Gain : Gain  Gain=8*1.875/1001
  Gain1 : Gain  Gain=100*(1+50/4.7)/2000
  Gain2 : Gain  Gain=100*(1+50/4.7)/2000
  Gain3 : Gain  Gain=8*1.875/1001
  Sum{,1..3} (4 alike) : Sum  Inputs=|++
  adc_interrup : Outport
  Vc : Outport  Port=2
  IL : Outport  Port=3
  Io : Outport  Port=4
  Vo_ADC : Outport  Port=5
  wires:
  Sum2/1 -> ADC Interface3/2
  adc_soc2/1 -> ADC Interface3/1
  ADC Interface3/2 -> Io/1
  Constant2/1 -> Sum2/2
  [I1] -> Gain2/1
  ADC Interface2/2 -> IL/1
  ADC Interface1/1 -> adc_interrup/1
  Constant1/1 -> Sum1/2
  Sum1/1 -> ADC Interface2/2
  [IL1] -> Gain1/1
  adc_soc1/1 -> ADC Interface2/1
  ADC Interface1/2 -> Vc/1
  Sum/1 -> ADC Interface1/2
  Constant/1 -> Sum/2
  [Vo1] -> Gain/1
  adc_soc/1 -> ADC Interface1/1
  Gain/1 -> Divide/1
  Gain1/1 -> Divide1/1
  Gain2/1 -> Divide2/1
  Divide2/1 -> Sum2/1
  Divide/1 -> Sum/1
  Divide1/1 -> Sum1/1
  Constant3/1 -> Divide/2
  Constant4/1 -> Divide1/2
  Constant5/1 -> Divide2/2
  Constant7/1 -> Divide3/2
  Constant6/1 -> Sum3/2
  Gain3/1 -> Divide3/1
  Divide3/1 -> Sum3/1
  ADC Interface4/2 -> Vo_ADC/1
  [Vo] -> Gain3/1
  adc_soc3/1 -> ADC Interface4/1
  Sum3/1 -> ADC Interface4/2

== system do_an_tn_ks/Message Triggered Subsystem/Bo dk ==
  err_vol : Inport
  IL1 : Inport  Port=2
  Vc1 : Inport  Port=3
  Enable : EnablePort
  Scope3 : Scope  NumInputPorts=2
  Sum : Sum  Inputs=|++
  Sum5 : Sum  Inputs=|+-
  curr_controller : Subsystem
  voltage_controller : Subsystem
  Out1 : Outport
  wires:
  Vc1/1 -> Sum/2
  Sum5/1 -> curr_controller/1(In1)
  curr_controller/1(Out1) -> Sum/1
  Sum/1 -> Out1/1
  err_vol/1 -> voltage_controller/1(In1)
  IL1/1 -> Scope3/2, Sum5/2
  voltage_controller/1(Out1) -> Scope3/1, Sum5/1

== system do_an_tn_ks/Message Triggered Subsystem/ConverADC ==
  Io_ADC : Inport
  Constant2 : Constant  Value=1.5*4096/3.3
  Constant9 : Constant  Value=sw1
  Current ADC Read - ADCC2 : prociolib/ADC Read  DataType=uint16  SampleTime=-1  NumCh=1  PeripheralConfigBtnCtrl=0  BlockSID=do_an_tn_ks:3536
  Data Type Conversion2 : DataTypeConversion  OutDataTypeStr=double  SaturateOnIntegerOverflow=off  RndMeth=Floor
  Gain3 : Gain  Gain=3.3*20/(4096*(1+50/4.7))
  Product : Product
  Sum1 : Sum  Inputs=|+-
  Io : Outport
  wires:
  Current ADC Read - ADCC2/1 -> Data Type Conversion2/1  "I_fbk"
  Data Type Conversion2/1 -> Sum1/1
  Constant9/1 -> Product/2
  Gain3/1 -> Product/1
  Constant2/1 -> Sum1/2
  Io_ADC/1 -> Current ADC Read - ADCC2/1
  Product/1 -> Io/1
  Sum1/1 -> Gain3/1

== system do_an_tn_ks/Message Triggered Subsystem/Pre_db ==
  V_ref1 : Inport
  Vo : Inport  Port=2
  Add : Sum  Inputs=+-
  Constant4 : Constant  Value=10
  Divide : Product  Inputs=*/
  Out1 : Outport
  wires:
  Add/1 -> Divide/1
  Vo/1 -> Add/2
  Constant4/1 -> Divide/2
  Divide/1 -> Out1/1
  V_ref1/1 -> Add/1

== system do_an_tn_ks/Message Triggered Subsystem/Subsystem ==
  Vo : Inport
  Vc1 : Inport  Port=2
  Inverter_OnOff : Inport  Port=3
  Abs : Abs  SaturateOnIntegerOverflow=off
  Abs1 : Abs  SaturateOnIntegerOverflow=off
  Chart1 : Stateflow chart  TreatAsAtomicUnit=on
      settings: PortSchema="{\"entries\":[{\"content\":{\"sides\":[{\"content\":{\"connectorIds\":[\"In4\",\"In3\",\"In1\",\"In2\"]},\"type\":\"ConnectorPlacement.EquallySpacedRectSide\",\"uuid\":\"a41d96ef-4339-445d-adf1-46a375c1ebfc\"},{\"content\":{\"connectorIds\":[\"Out1\",\"Out2\"],\"side\":\"RIGHT\"},\"type\":\"ConnectorPlacement.EquallySpacedRectSide\",\"uuid\":\"433b8e1f-da11-4860-b5b3-686501ffdddb\"},{\"content\":{\"side\":\"TOP\"},\"type\":\"ConnectorPlacement.EquallySpacedRectSide\",\"uuid\":\"a76241af-ec7f-4a92-ba0a-9793b7afdcf0\"}]},\"type\":\"ConnectorPlacement.EquallySpacedConnector\",\"uuid\":\"1de099f0-7c57-4924-8764-8a627297889a\"}],\"packageUris\":[\"http://schema.mathworks.com/mf0/Connector/R2020b\"],\"version\":\"1.0\"}"
  MATLAB Function : MATLAB Function  TreatAsAtomicUnit=on
  MATLAB Function1 : MATLAB Function  TreatAsAtomicUnit=on
  Scope6 : Scope
  Sum6 : Sum  Inputs=|+-
  Terminator : Terminator
  Terminator1 : Terminator
  En_Relay : Outport
  enable_bdk : Outport  Port=2
  wires:
  MATLAB Function/1(Vrms) -> Chart1/3(Vout_Rms), Sum6/1
  MATLAB Function1/2(theta) -> Terminator/1
  MATLAB Function/2(theta) -> Terminator1/1
  MATLAB Function1/1(Vrms) -> Sum6/2
  Abs1/1 -> Chart1/1(Error_RMS)
  Vc1/1 -> Abs/1, MATLAB Function1/1(vin)
  Sum6/1 -> Abs1/1, Scope6/1
  Abs/1 -> Chart1/4(Vc1_abs)
  Inverter_OnOff/1 -> Chart1/2(Inverter_OnOff)
  Chart1/1(En_Relay) -> En_Relay/1
  Vo/1 -> MATLAB Function/1(vin)
  Chart1/2(enable_bdk) -> enable_bdk/1

== system do_an_tn_ks/Message Triggered Subsystem/Subsystem1 ==
  Vo_ADC : Inport
  Constant5 : Constant  Value=1.5*4096/3.3
  Constant6 : Constant  Value=sw
  Current ADC Read - ADCC3 : prociolib/ADC Read  DataType=uint16  SampleTime=-1  NumCh=1  PeripheralConfigBtnCtrl=0  BlockSID=do_an_tn_ks:3953
  Data Type Conversion3 : DataTypeConversion  OutDataTypeStr=double  SaturateOnIntegerOverflow=off  RndMeth=Floor
  Gain4 : Gain  Gain=3.3*1001/(8*4096*1.875)
  Product2 : Product
  Sum8 : Sum  Inputs=|+-
  Vo : Outport
  wires:
  Sum8/1 -> Gain4/1
  Constant5/1 -> Sum8/2
  Current ADC Read - ADCC3/1 -> Data Type Conversion3/1  "I_fbk"
  Gain4/1 -> Product2/1
  Product2/1 -> Vo/1
  Data Type Conversion3/1 -> Sum8/1
  Vo_ADC/1 -> Current ADC Read - ADCC3/1
  Constant6/1 -> Product2/2

== system do_an_tn_ks/Message Triggered Subsystem/Subsystem2 ==
  Vc_ADC : Inport
  Constant : Constant  Value=1.5*4096/3.3
  Constant7 : Constant  Value=sw
  Current ADC Read - ADCC5 : prociolib/ADC Read  DataType=uint16  SampleTime=-1  NumCh=1  PeripheralConfigBtnCtrl=0  BlockSID=do_an_tn_ks:3404
  Data Type Conversion : DataTypeConversion  OutDataTypeStr=double  SaturateOnIntegerOverflow=off  RndMeth=Floor
  Gain13 : Gain  Gain=3.3*1001/(8*4096*1.875)
  Product3 : Product
  Sum2 : Sum  Inputs=|+-
  Vc : Outport
  wires:
  Gain13/1 -> Product3/1
  Current ADC Read - ADCC5/1 -> Data Type Conversion/1  "I_fbk"
  Sum2/1 -> Gain13/1
  Product3/1 -> Vc/1
  Constant/1 -> Sum2/2
  Vc_ADC/1 -> Current ADC Read - ADCC5/1
  Data Type Conversion/1 -> Sum2/1
  Constant7/1 -> Product3/2

== system do_an_tn_ks/Message Triggered Subsystem/Subsystem3 ==
  IL_ADC : Inport
  Constant3 : Constant  Value=1.5*4096/3.3
  Constant8 : Constant  Value=sw1
  Current ADC Read - ADCC1 : prociolib/ADC Read  DataType=uint16  SampleTime=-1  NumCh=1  PeripheralConfigBtnCtrl=0  BlockSID=do_an_tn_ks:3403
  Data Type Conversion1 : DataTypeConversion  OutDataTypeStr=double  SaturateOnIntegerOverflow=off  RndMeth=Floor
  Gain14 : Gain  Gain=3.3*20/(4096*(1+50/4.7))
  Product4 : Product
  Sum4 : Sum  Inputs=|+-
  IL : Outport
  wires:
  Current ADC Read - ADCC1/1 -> Data Type Conversion1/1  "I_fbk"
  Product4/1 -> IL/1
  Gain14/1 -> Product4/1
  Sum4/1 -> Gain14/1
  Constant3/1 -> Sum4/2
  Data Type Conversion1/1 -> Sum4/1
  Constant8/1 -> Product4/2
  IL_ADC/1 -> Current ADC Read - ADCC1/1

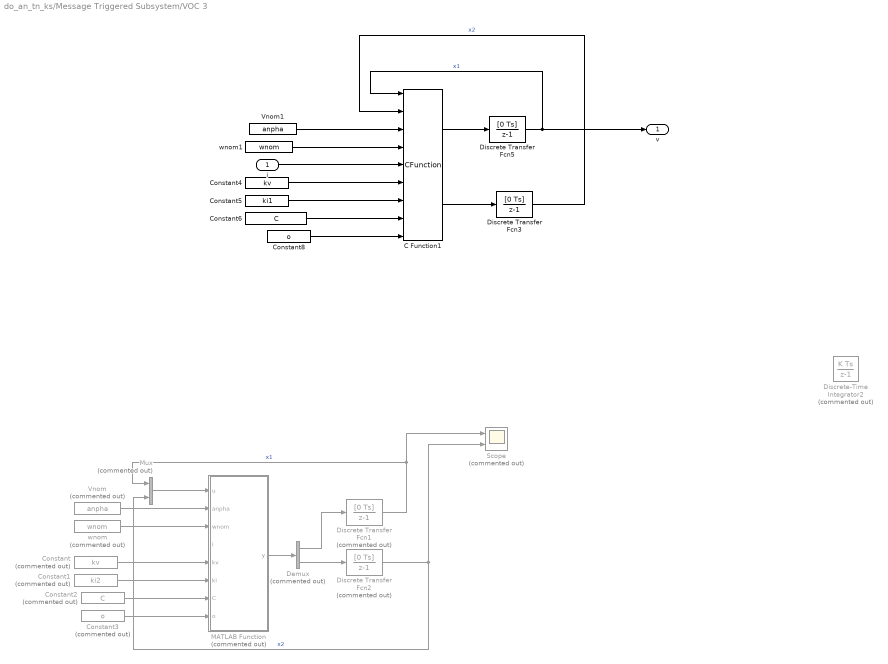
== system do_an_tn_ks/Message Triggered Subsystem/VOC 3 ==
  i : Inport
  C Function1 : CFunction  OutputCode=|
      | y1 = (kv*kv*o/anpha-u1*u1-u2*u2)*u1*anpha/(C*kv*kv)-wnom*u2-ki*kv*i/C;
      | y2 = wnom*u1;
  Constant : Constant  Commented=on  Value=kv  OutDataTypeStr=double  SampleTime=-1
  Constant1 : Constant  Commented=on  Value=ki2  OutDataTypeStr=double  SampleTime=-1
  Constant2 : Constant  Commented=on  Value=C  OutDataTypeStr=double  SampleTime=-1
  Constant3 : Constant  Commented=on  Value=o  OutDataTypeStr=double  SampleTime=-1
  Constant4 : Constant  Value=kv  OutDataTypeStr=double  SampleTime=-1
  Constant5 : Constant  Value=ki1  OutDataTypeStr=double  SampleTime=-1
  Constant6 : Constant  Value=C  OutDataTypeStr=double  SampleTime=-1
  Constant8 : Constant  Value=o  OutDataTypeStr=double  SampleTime=-1
  Demux : Demux  Commented=on  Outputs=2
  Discrete Transfer Fcn1 : DiscreteTransferFcn  Commented=on  Numerator=[0 Ts]  Denominator=[1 -1]  SampleTime=Ts
  Discrete Transfer Fcn2 : DiscreteTransferFcn  Commented=on  Numerator=[0 Ts]  Denominator=[1 -1]  SampleTime=Ts
  Discrete Transfer Fcn3 : DiscreteTransferFcn  Numerator=[0 Ts]  Denominator=[1 -1]
  Discrete Transfer Fcn5 : DiscreteTransferFcn  Numerator=[0 Ts]  Denominator=[1 -1]
  Discrete-Time Integrator2 : DiscreteIntegrator  Commented=on  InitialCondition=0.5  SampleTime=Ts  ICPrevOutput=DiscIntNeverNeededParam  ICPrevScaledInput=DiscIntNeverNeededParam
  MATLAB Function : MATLAB Function  Commented=on  TreatAsAtomicUnit=on
  Mux : Mux  Commented=on  Inputs=2
  Scope : Scope  Commented=on  NumInputPorts=2
  Vnom : Constant  Commented=on  Value=anpha  OutDataTypeStr=double  SampleTime=-1
  Vnom1 : Constant  Value=anpha  OutDataTypeStr=double  SampleTime=-1
  wnom : Constant  Commented=on  Value=wnom  OutDataTypeStr=double  SampleTime=-1
  wnom1 : Constant  Value=wnom  OutDataTypeStr=double  SampleTime=-1
  v : Outport
  wires:
  wnom/1 -> MATLAB Function/3(wnom)
  Discrete Transfer Fcn1/1 -> Scope/1, Mux/1  "x1"
  Mux/1 -> MATLAB Function/1(u)
  Demux/2 -> Discrete Transfer Fcn2/1
  MATLAB Function/1(y) -> Demux/1
  Demux/1 -> Discrete Transfer Fcn1/1
  Discrete Transfer Fcn2/1 -> Scope/2, Mux/2  "x2"
  Vnom/1 -> MATLAB Function/2(anpha)
  Constant/1 -> MATLAB Function/5(kv)
  Constant1/1 -> MATLAB Function/6(ki)
  Constant2/1 -> MATLAB Function/7(C)
  Constant3/1 -> MATLAB Function/8(o)
  Discrete Transfer Fcn5/1 -> C Function1/1, v/1  "x1"
  C Function1/1 -> Discrete Transfer Fcn5/1
  Vnom1/1 -> C Function1/3
  Constant8/1 -> C Function1/9
  Constant4/1 -> C Function1/6
  Constant6/1 -> C Function1/8
  C Function1/2 -> Discrete Transfer Fcn3/1
  wnom1/1 -> C Function1/4
  Constant5/1 -> C Function1/7
  Discrete Transfer Fcn3/1 -> C Function1/2  "x2"
  i/1 -> C Function1/5

== system do_an_tn_ks/Message Triggered Subsystem1/ConverADC ==
  Io_ADC : Inport
  Constant2 : Constant  Value=1.5*4096/3.3
  Constant9 : Constant  Value=sw1
  Current ADC Read - ADCC2 : prociolib/ADC Read  DataType=uint16  SampleTime=-1  NumCh=1  PeripheralConfigBtnCtrl=0  BlockSID=do_an_tn_ks:4141
  Data Type Conversion2 : DataTypeConversion  OutDataTypeStr=double  SaturateOnIntegerOverflow=off  RndMeth=Floor
  Gain3 : Gain  Gain=3.3*20/(4096*(1+50/4.7))
  Product : Product
  Sum1 : Sum  Inputs=|+-
  Io : Outport
  wires:
  Sum1/1 -> Gain3/1
  Product/1 -> Io/1
  Io_ADC/1 -> Current ADC Read - ADCC2/1
  Constant2/1 -> Sum1/2
  Gain3/1 -> Product/1
  Constant9/1 -> Product/2
  Data Type Conversion2/1 -> Sum1/1
  Current ADC Read - ADCC2/1 -> Data Type Conversion2/1  "I_fbk"

== system do_an_tn_ks/Message Triggered Subsystem1/Pre_db ==
  V_ref1 : Inport
  Vo : Inport  Port=2
  Add : Sum  Inputs=+-
  Constant4 : Constant  Value=10
  Divide : Product  Inputs=*/
  Out1 : Outport
  wires:
  V_ref1/1 -> Add/1
  Divide/1 -> Out1/1
  Constant4/1 -> Divide/2
  Vo/1 -> Add/2
  Add/1 -> Divide/1

== system do_an_tn_ks/Message Triggered Subsystem1/Subsystem ==
  Vo : Inport
  Vc1 : Inport  Port=2
  Inverter_OnOff : Inport  Port=3
  Abs : Abs  SaturateOnIntegerOverflow=off
  Abs1 : Abs  SaturateOnIntegerOverflow=off
  Chart1 : Stateflow chart  TreatAsAtomicUnit=on
      settings: PortSchema="{\"entries\":[{\"content\":{\"sides\":[{\"content\":{\"connectorIds\":[\"In4\",\"In3\",\"In1\",\"In2\"]},\"type\":\"ConnectorPlacement.EquallySpacedRectSide\",\"uuid\":\"a41d96ef-4339-445d-adf1-46a375c1ebfc\"},{\"content\":{\"connectorIds\":[\"Out1\",\"Out2\"],\"side\":\"RIGHT\"},\"type\":\"ConnectorPlacement.EquallySpacedRectSide\",\"uuid\":\"433b8e1f-da11-4860-b5b3-686501ffdddb\"},{\"content\":{\"side\":\"TOP\"},\"type\":\"ConnectorPlacement.EquallySpacedRectSide\",\"uuid\":\"a76241af-ec7f-4a92-ba0a-9793b7afdcf0\"}]},\"type\":\"ConnectorPlacement.EquallySpacedConnector\",\"uuid\":\"1de099f0-7c57-4924-8764-8a627297889a\"}],\"packageUris\":[\"http://schema.mathworks.com/mf0/Connector/R2020b\"],\"version\":\"1.0\"}"
  MATLAB Function : MATLAB Function  TreatAsAtomicUnit=on
  MATLAB Function1 : MATLAB Function  TreatAsAtomicUnit=on
  Scope6 : Scope
  Sum6 : Sum  Inputs=|+-
  Terminator : Terminator
  Terminator1 : Terminator
  En_Relay : Outport
  enable_bdk : Outport  Port=2
  wires:
  Chart1/2(enable_bdk) -> enable_bdk/1
  Vo/1 -> MATLAB Function/1(vin)
  Chart1/1(En_Relay) -> En_Relay/1
  Inverter_OnOff/1 -> Chart1/2(Inverter_OnOff)
  Abs/1 -> Chart1/4(Vc1_abs)
  Sum6/1 -> Scope6/1, Abs1/1
  Vc1/1 -> MATLAB Function1/1(vin), Abs/1
  Abs1/1 -> Chart1/1(Error_RMS)
  MATLAB Function1/1(Vrms) -> Sum6/2
  MATLAB Function/2(theta) -> Terminator1/1
  MATLAB Function1/2(theta) -> Terminator/1
  MATLAB Function/1(Vrms) -> Sum6/1, Chart1/3(Vout_Rms)

== system do_an_tn_ks/Message Triggered Subsystem1/Subsystem1 ==
  Vo_ADC : Inport
  Constant5 : Constant  Value=1.5*4096/3.3
  Constant6 : Constant  Value=sw
  Current ADC Read - ADCC3 : prociolib/ADC Read  DataType=uint16  SampleTime=-1  NumCh=1  PeripheralConfigBtnCtrl=0  BlockSID=do_an_tn_ks:4202
  Data Type Conversion3 : DataTypeConversion  OutDataTypeStr=double  SaturateOnIntegerOverflow=off  RndMeth=Floor
  Gain4 : Gain  Gain=3.3*1001/(8*4096*1.875)
  Product2 : Product
  Sum8 : Sum  Inputs=|+-
  Vo : Outport
  wires:
  Constant6/1 -> Product2/2
  Vo_ADC/1 -> Current ADC Read - ADCC3/1
  Data Type Conversion3/1 -> Sum8/1
  Product2/1 -> Vo/1
  Gain4/1 -> Product2/1
  Current ADC Read - ADCC3/1 -> Data Type Conversion3/1  "I_fbk"
  Constant5/1 -> Sum8/2
  Sum8/1 -> Gain4/1

== system do_an_tn_ks/Message Triggered Subsystem1/Subsystem2 ==
  Vc_ADC : Inport
  Constant : Constant  Value=1.5*4096/3.3
  Constant7 : Constant  Value=sw
  Current ADC Read - ADCC5 : prociolib/ADC Read  DataType=uint16  SampleTime=-1  NumCh=1  PeripheralConfigBtnCtrl=0  BlockSID=do_an_tn_ks:4212
  Data Type Conversion : DataTypeConversion  OutDataTypeStr=double  SaturateOnIntegerOverflow=off  RndMeth=Floor
  Gain13 : Gain  Gain=3.3*1001/(8*4096*1.875)
  Product3 : Product
  Sum2 : Sum  Inputs=|+-
  Vc : Outport
  wires:
  Constant7/1 -> Product3/2
  Data Type Conversion/1 -> Sum2/1
  Vc_ADC/1 -> Current ADC Read - ADCC5/1
  Constant/1 -> Sum2/2
  Product3/1 -> Vc/1
  Sum2/1 -> Gain13/1
  Current ADC Read - ADCC5/1 -> Data Type Conversion/1  "I_fbk"
  Gain13/1 -> Product3/1

== system do_an_tn_ks/Message Triggered Subsystem1/Subsystem3 ==
  IL_ADC : Inport
  Constant3 : Constant  Value=1.5*4096/3.3
  Constant8 : Constant  Value=sw1
  Current ADC Read - ADCC1 : prociolib/ADC Read  DataType=uint16  SampleTime=-1  NumCh=1  PeripheralConfigBtnCtrl=0  BlockSID=do_an_tn_ks:4222
  Data Type Conversion1 : DataTypeConversion  OutDataTypeStr=double  SaturateOnIntegerOverflow=off  RndMeth=Floor
  Gain14 : Gain  Gain=3.3*20/(4096*(1+50/4.7))
  Product4 : Product
  Sum4 : Sum  Inputs=|+-
  IL : Outport
  wires:
  IL_ADC/1 -> Current ADC Read - ADCC1/1
  Constant8/1 -> Product4/2
  Data Type Conversion1/1 -> Sum4/1
  Constant3/1 -> Sum4/2
  Sum4/1 -> Gain14/1
  Gain14/1 -> Product4/1
  Product4/1 -> IL/1
  Current ADC Read - ADCC1/1 -> Data Type Conversion1/1  "I_fbk"

== system do_an_tn_ks/Message Triggered Subsystem1/Subsystem4 ==
  err_vol : Inport
  IL1 : Inport  Port=2
  Vc1 : Inport  Port=3
  Enable : EnablePort
  Scope3 : Scope  NumInputPorts=2
  Sum : Sum  Inputs=|++
  Sum5 : Sum  Inputs=|+-
  curr_controller : Subsystem
  voltage_controller : Subsystem
  Out1 : Outport
  wires:
  voltage_controller/1(Out1) -> Sum5/1, Scope3/1
  IL1/1 -> Sum5/2, Scope3/2
  err_vol/1 -> voltage_controller/1(In1)
  Sum/1 -> Out1/1
  curr_controller/1(Out1) -> Sum/1
  Sum5/1 -> curr_controller/1(In1)
  Vc1/1 -> Sum/2

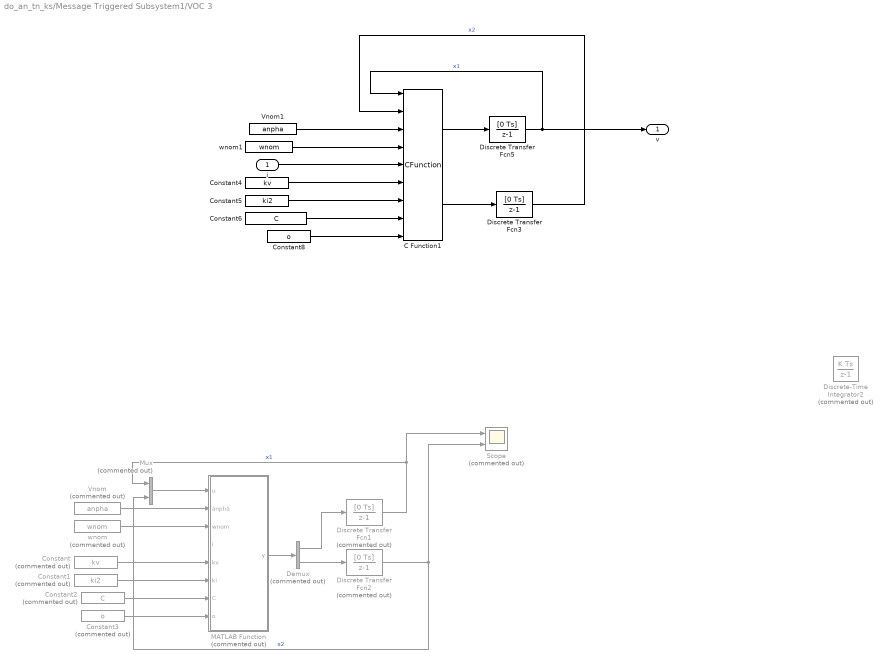
== system do_an_tn_ks/Message Triggered Subsystem1/VOC 3 ==
  i : Inport
  C Function1 : CFunction  OutputCode=|
      | y1 = (kv*kv*o/anpha-u1*u1-u2*u2)*u1*anpha/(C*kv*kv)-wnom*u2-ki*kv*i/C;
      | y2 = wnom*u1;
  Constant : Constant  Commented=on  Value=kv  OutDataTypeStr=double  SampleTime=-1
  Constant1 : Constant  Commented=on  Value=ki2  OutDataTypeStr=double  SampleTime=-1
  Constant2 : Constant  Commented=on  Value=C  OutDataTypeStr=double  SampleTime=-1
  Constant3 : Constant  Commented=on  Value=o  OutDataTypeStr=double  SampleTime=-1
  Constant4 : Constant  Value=kv  OutDataTypeStr=double  SampleTime=-1
  Constant5 : Constant  Value=ki2  OutDataTypeStr=double  SampleTime=-1
  Constant6 : Constant  Value=C  OutDataTypeStr=double  SampleTime=-1
  Constant8 : Constant  Value=o  OutDataTypeStr=double  SampleTime=-1
  Demux : Demux  Commented=on  Outputs=2
  Discrete Transfer Fcn1 : DiscreteTransferFcn  Commented=on  Numerator=[0 Ts]  Denominator=[1 -1]  SampleTime=Ts
  Discrete Transfer Fcn2 : DiscreteTransferFcn  Commented=on  Numerator=[0 Ts]  Denominator=[1 -1]  SampleTime=Ts
  Discrete Transfer Fcn3 : DiscreteTransferFcn  Numerator=[0 Ts]  Denominator=[1 -1]
  Discrete Transfer Fcn5 : DiscreteTransferFcn  Numerator=[0 Ts]  Denominator=[1 -1]
  Discrete-Time Integrator2 : DiscreteIntegrator  Commented=on  InitialCondition=0.5  SampleTime=Ts  ICPrevOutput=DiscIntNeverNeededParam  ICPrevScaledInput=DiscIntNeverNeededParam
  MATLAB Function : MATLAB Function  Commented=on  TreatAsAtomicUnit=on
  Mux : Mux  Commented=on  Inputs=2
  Scope : Scope  Commented=on  NumInputPorts=2
  Vnom : Constant  Commented=on  Value=anpha  OutDataTypeStr=double  SampleTime=-1
  Vnom1 : Constant  Value=anpha  OutDataTypeStr=double  SampleTime=-1
  wnom : Constant  Commented=on  Value=wnom  OutDataTypeStr=double  SampleTime=-1
  wnom1 : Constant  Value=wnom  OutDataTypeStr=double  SampleTime=-1
  v : Outport
  wires:
  i/1 -> C Function1/5
  Discrete Transfer Fcn3/1 -> C Function1/2  "x2"
  Constant5/1 -> C Function1/7
  wnom1/1 -> C Function1/4
  C Function1/2 -> Discrete Transfer Fcn3/1
  Constant6/1 -> C Function1/8
  Constant4/1 -> C Function1/6
  Constant8/1 -> C Function1/9
  Vnom1/1 -> C Function1/3
  C Function1/1 -> Discrete Transfer Fcn5/1
  Discrete Transfer Fcn5/1 -> v/1, C Function1/1  "x1"
  Constant3/1 -> MATLAB Function/8(o)
  Constant2/1 -> MATLAB Function/7(C)
  Constant1/1 -> MATLAB Function/6(ki)
  Constant/1 -> MATLAB Function/5(kv)
  Vnom/1 -> MATLAB Function/2(anpha)
  Discrete Transfer Fcn2/1 -> Mux/2, Scope/2  "x2"
  Demux/1 -> Discrete Transfer Fcn1/1
  MATLAB Function/1(y) -> Demux/1
  Demux/2 -> Discrete Transfer Fcn2/1
  Mux/1 -> MATLAB Function/1(u)
  Discrete Transfer Fcn1/1 -> Mux/1, Scope/1  "x1"
  wnom/1 -> MATLAB Function/3(wnom)
